simulink model "MdEnChk6s7s_LugL"  (R2018b)
settings: Solver=FixedStepDiscrete  StartTime=0.0  StopTime=10.0  FixedStep=0.01  RelTol=1e-3
settings Model: Creator=sn2xws  LastModifiedBy=sn2xws
settings DataIOCC: SaveFormat=StructureWithTime
settings OptimizationCC: DefaultParameterBehavior=Inlined  EnhancedBackFolding=on  PassReuseOutputArgsAs=Individual arguments  ZeroExternalMemoryAtStartup=off  ZeroInternalMemoryAtStartup=off  OptimizeBlockOrder=speed  DifferentSizesBufferReuse=on  OptimizationCustomize=off
settings DebuggingCC: ParameterTunabilityLossMsg=error
settings ModelReferenceCC: ModelReferenceNumInstancesAllowed=Single
settings SFSimCC: MATLABDynamicMemAlloc=off
settings RTWCC: SystemTargetFile=autosar.tlc  GenCodeOnly=on  TemplateMakefile=ert_default_tmf  Description=AUTOSAR  GenerateReport=on  IncludeHyperlinkInReport=on  LaunchReport=on  GenerateTraceInfo=on  GenerateTraceReport=on  GenerateTraceReportSl=on  GenerateTraceReportSf=on  GenerateTraceReportEml=on
settings CodeAppCC: ForceParamTrailComments=on  IgnoreCustomStorageClasses=off  OperatorAnnotations=on  SimulinkDataObjDesc=on  SFDataObjDesc=on  InsertBlockDesc=on
settings STFCustomTargetCC: TargetLangStandard=C99 (ISO)  MultiwordLength=256  ParMdlRefBuildCompliant=on  CompOptLevelCompliant=on  IncludeMdlTerminateFcn=off  CombineOutputUpdateFcns=on  SuppressErrorStatus=on  ERTCustomFileBanners=on  SupportNonFinite=off  SupportComplex=off  SupportContinuousTime=off  SupportNonInlinedSFcns=off  RemoveResetFunc=on  MATLABClassNameForMDSCustomization=Simulink.SoftwareTarget.ERTCustomization  AutosarCompliant=on  UseToolchainInfoCompliant=on  LookupTableObjectStructAxisOrder=2,1,3,4,...  LUTObjectStructOrderEvenSpacing=Size,Table,Breakpoints  SystemTargetFile=autosar.tlc
settings ERTTargetCC: TargetLangStandard=C99 (ISO)  ConcurrentExecutionCompliant=off  IncludeMdlTerminateFcn=off  SuppressErrorStatus=on  SupportNonFinite=off  SupportComplex=off  ModelStepFunctionPrototypeControlCompliant=off  CPPClassGenCompliant=off  AutosarCompliant=on  LookupTableObjectStructAxisOrder=2,1,3,4,...  LUTObjectStructOrderEvenSpacing=Size,Table,Breakpoints  InlinedParameterPlacement=NonHierarchical  ERTCustomFileTemplate=example_file_process.tlc

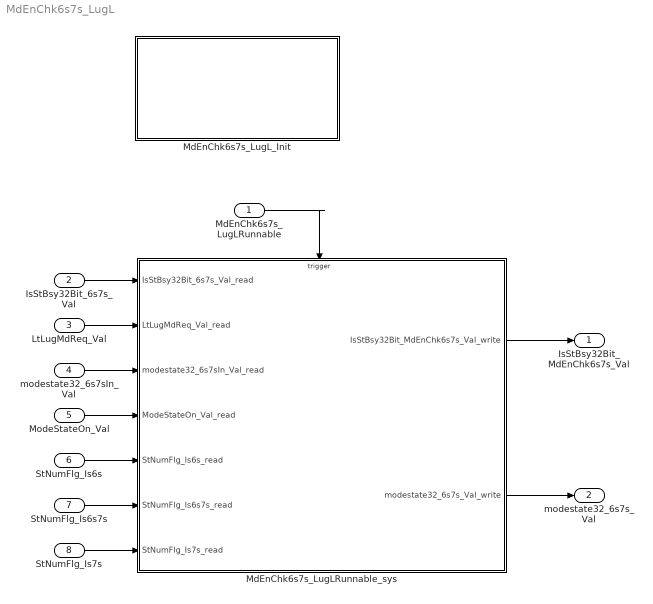
== system MdEnChk6s7s_LugL ==
  MdEnChk6s7s_LugLRunnable : Inport  SampleTime=0.01  OutputFunctionCall=on
  IsStBsy32Bit_6s7s_Val : Inport  Port=2  OutDataTypeStr=uint32  PortDimensions=1
  LtLugMdReq_Val : Inport  Port=3  OutDataTypeStr=boolean  PortDimensions=1
  modestate32_6s7sIn_Val : Inport  Port=4  OutDataTypeStr=uint32  PortDimensions=1
  ModeStateOn_Val : Inport  Port=5  OutDataTypeStr=boolean  PortDimensions=1
  StNumFlg_Is6s : Inport  Port=6  OutDataTypeStr=boolean  PortDimensions=1
  StNumFlg_Is6s7s : Inport  Port=7  OutDataTypeStr=boolean  PortDimensions=1
  StNumFlg_Is7s : Inport  Port=8  OutDataTypeStr=boolean  PortDimensions=1
  MdEnChk6s7s_LugLRunnable_sys : Subsystem
  MdEnChk6s7s_LugL_Init : Subsystem
  IsStBsy32Bit_MdEnChk6s7s_Val : Outport  OutDataTypeStr=uint32  PortDimensions=1
  modestate32_6s7s_Val : Outport  Port=2  OutDataTypeStr=uint32  PortDimensions=1
  wires:
  IsStBsy32Bit_6s7s_Val/1 -> MdEnChk6s7s_LugLRunnable_sys/1(IsStBsy32Bit_6s7s_Val_read)
  LtLugMdReq_Val/1 -> MdEnChk6s7s_LugLRunnable_sys/2(LtLugMdReq_Val_read)
  modestate32_6s7sIn_Val/1 -> MdEnChk6s7s_LugLRunnable_sys/3(modestate32_6s7sIn_Val_read)
  ModeStateOn_Val/1 -> MdEnChk6s7s_LugLRunnable_sys/4(ModeStateOn_Val_read)
  StNumFlg_Is6s/1 -> MdEnChk6s7s_LugLRunnable_sys/5(StNumFlg_Is6s_read)
  StNumFlg_Is6s7s/1 -> MdEnChk6s7s_LugLRunnable_sys/6(StNumFlg_Is6s7s_read)
  StNumFlg_Is7s/1 -> MdEnChk6s7s_LugLRunnable_sys/7(StNumFlg_Is7s_read)
  MdEnChk6s7s_LugLRunnable_sys/1(IsStBsy32Bit_MdEnChk6s7s_Val_write) -> IsStBsy32Bit_MdEnChk6s7s_Val/1
  MdEnChk6s7s_LugLRunnable_sys/2(modestate32_6s7s_Val_write) -> modestate32_6s7s_Val/1
  MdEnChk6s7s_LugLRunnable/1 -> MdEnChk6s7s_LugLRunnable_sys/Trigger

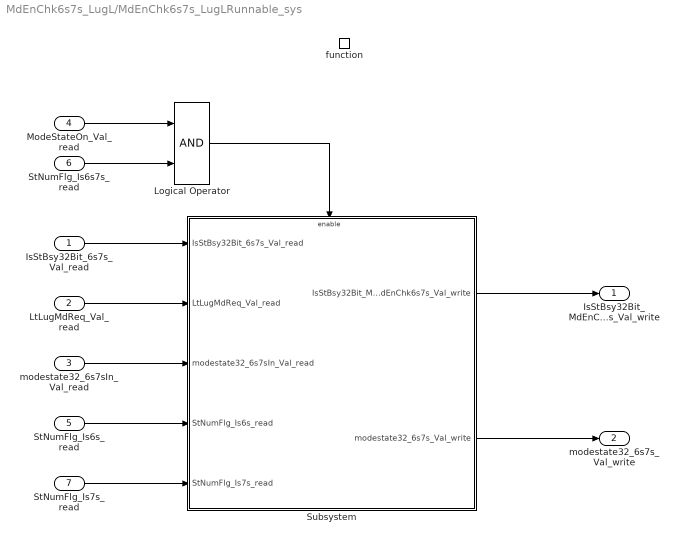
== system MdEnChk6s7s_LugL/MdEnChk6s7s_LugLRunnable_sys ==
  IsStBsy32Bit_6s7s_Val_read : Inport
  LtLugMdReq_Val_read : Inport  Port=2
  modestate32_6s7sIn_Val_read : Inport  Port=3
  ModeStateOn_Val_read : Inport  Port=4
  StNumFlg_Is6s_read : Inport  Port=5
  StNumFlg_Is6s7s_read : Inport  Port=6
  StNumFlg_Is7s_read : Inport  Port=7
  function : TriggerPort  TriggerType=function-call  VariantControl=(inherit)  SampleTimeType=periodic  SampleTime=-1
  Logical Operator : Logic  AllPortsSameDT=off  OutDataTypeStr=boolean
  Subsystem : Subsystem
  IsStBsy32Bit_MdEnChk6s7s_Val_write : Outport
      settings: EnsureOutportIsVirtual=on
  modestate32_6s7s_Val_write : Outport  Port=2
      settings: EnsureOutportIsVirtual=on
  wires:
  IsStBsy32Bit_6s7s_Val_read/1 -> Subsystem/1(IsStBsy32Bit_6s7s_Val_read)
  LtLugMdReq_Val_read/1 -> Subsystem/2(LtLugMdReq_Val_read)
  modestate32_6s7sIn_Val_read/1 -> Subsystem/3(modestate32_6s7sIn_Val_read)
  StNumFlg_Is6s_read/1 -> Subsystem/4(StNumFlg_Is6s_read)
  StNumFlg_Is7s_read/1 -> Subsystem/5(StNumFlg_Is7s_read)
  Subsystem/1(IsStBsy32Bit_MdEnChk6s7s_Val_write) -> IsStBsy32Bit_MdEnChk6s7s_Val_write/1
  Subsystem/2(modestate32_6s7s_Val_write) -> modestate32_6s7s_Val_write/1
  StNumFlg_Is6s7s_read/1 -> Logical Operator/2
  Logical Operator/1 -> Subsystem/Enable
  ModeStateOn_Val_read/1 -> Logical Operator/1

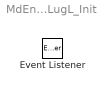
== system MdEnChk6s7s_LugL/MdEnChk6s7s_LugL_Init ==
  Event Listener : EventListener  EventName=reset

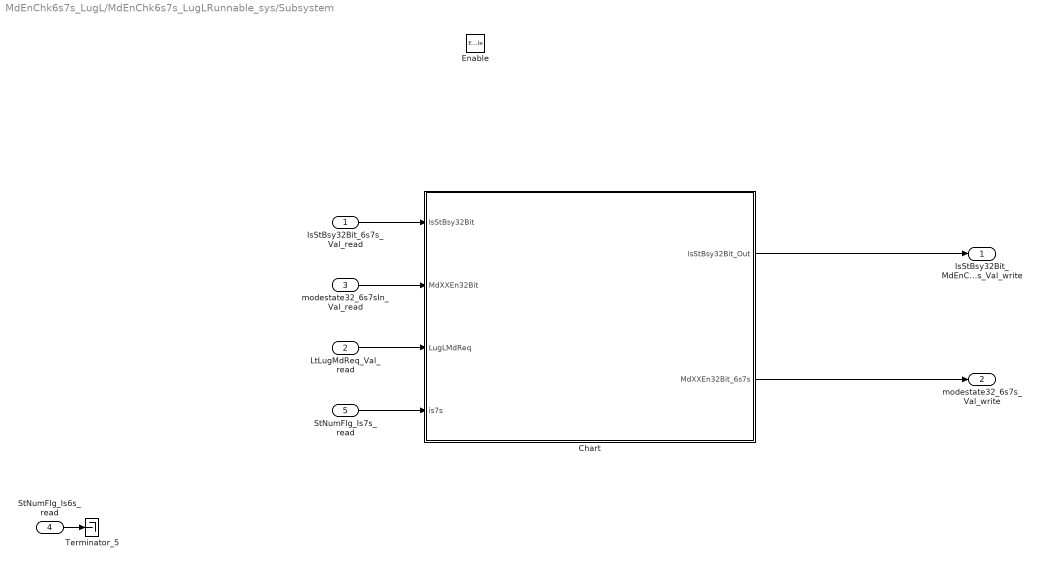
== system MdEnChk6s7s_LugL/MdEnChk6s7s_LugLRunnable_sys/Subsystem ==
  IsStBsy32Bit_6s7s_Val_read : Inport
  LtLugMdReq_Val_read : Inport  Port=2
  modestate32_6s7sIn_Val_read : Inport  Port=3
  StNumFlg_Is6s_read : Inport  Port=4
  StNumFlg_Is7s_read : Inport  Port=5
  Enable : EnablePort
  Chart : Stateflow chart  TreatAsAtomicUnit=on
  Terminator_5 : Terminator
  IsStBsy32Bit_MdEnChk6s7s_Val_write : Outport
      settings: EnsureOutportIsVirtual=on
  modestate32_6s7s_Val_write : Outport  Port=2
      settings: EnsureOutportIsVirtual=on
  wires:
  StNumFlg_Is7s_read/1 -> Chart/4(is7s)
  Chart/1(IsStBsy32Bit_Out) -> IsStBsy32Bit_MdEnChk6s7s_Val_write/1
  StNumFlg_Is6s_read/1 -> Terminator_5/1
  IsStBsy32Bit_6s7s_Val_read/1 -> Chart/1(IsStBsy32Bit)
  Chart/2(MdXXEn32Bit_6s7s) -> modestate32_6s7s_Val_write/1
  LtLugMdReq_Val_read/1 -> Chart/3(LugLMdReq)
  modestate32_6s7sIn_Val_read/1 -> Chart/2(MdXXEn32Bit)

== stateflow chart MdEnChk6s7s_LugL/MdEnChk6s7s_LugLRunnable_sys/Subsystem/Chart ==
  state LftMdBsySet6s7s [function]
    (default) -> (junction 191)
    (junction 191) -> (junction 192) : {
        | IsStBsy32Bit_Out = IsStBsy32Bit_Out|(EZEBit+EZQBit+VIPLBit+VIPAllBit+RcvyLBit+LugLBit+LugAllBit+FamlyLBit+FamlyRBit+INTMLBit+INTMRBit);
        | }
    (junction 192) -> (junction 193)
  (default) -> (junction 33) : {
      | IsStBsy32Bit_Out =IsStBsy32Bit;
      | MdXXEn32Bit_6s7s = MdXXEn32Bit;
      | }
  (junction 33) -> (junction 37) [order 1] : [hasChangedTo(LugLMdReq,true)&&((MdXXEn32Bit_6s7s&LugLBit)==0)]
  (junction 33) -> (junction 40) [order 2]
  (junction 37) -> (junction 39) : {
      | MdXXEn32Bit_6s7s=MdXXEn32Bit_6s7s|LugLBit;
      | LftMdBsySet6s7s();
      | IsStBsy32Bit_Out = IsStBsy32Bit_Out|(is7s<<12);/*RcvyRBit*/
      | IsStBsy32Bit_Out = IsStBsy32Bit_Out|(is7s<<11);/*VIPRBit*/
      | }
  (junction 39) -> (junction 40)
  (junction 40) -> (junction 247)
  data: IsStBsy32Bit_Out output uint32; MdXXEn32Bit_6s7s output uint32; IsStBsy32Bit input uint32; MdXXEn32Bit input uint32; EZEBit constant uint32 =1; EZQBit constant uint32 =8; VIPAllBit constant uint32 =2; LugAllBit constant uint32 =4; VIPLBit constant uint32 =512; RcvyLBit constant uint32 =1024; INTMLBit constant uint32 =16; INTMRBit constant uint32 =524288; FamlyLBit constant uint32 =64; FamlyRBit constant uint32 =32; LugLBit constant uint32 =128; LugLMdReq input; is7s input
